simulink library "csu_mhn_miru_hardware_noise_lib"  (R2015b)
settings: Solver=ode45  SolverMode=SingleTasking  StartTime=0.0  StopTime=10.0  RelTol=1e-3
values from neighbouring files (symbols this model uses):
  mhn_accel_range = 3*9.81    (= 29.43)    [csu_mhn_miru_hardware_noise_init.m]
  mhn_accel_SF = 300/1e6    (= 0.0003)    [csu_mhn_miru_hardware_noise_init.m]
  mhn_correlation_time = 100    [csu_mhn_miru_hardware_noise_init.m]
  mhn_dt = sim_time_step_size    [csu_mhn_miru_hardware_noise_init.m]
  mhn_gyro_g_sensitive = 2.471e-08 * [1 1 1]'    [csu_mhn_miru_hardware_noise_init.m]
  mhn_gyro_range = 250*pi/180    (= 4.36332312999)    [csu_mhn_miru_hardware_noise_init.m]
  mhn_gyro_SF = 100/1e6    (= 0.0001)    [csu_mhn_miru_hardware_noise_init.m]
  mhn_gyro_vibe_sensitive = 5.04e-09 * [1 1 1]'    [csu_mhn_miru_hardware_noise_init.m]
libraries: util_common_lib x7, util_info_lib x1
settings Model: Creator=hcannon  LastModifiedBy=Mark Agbayani
settings DataIOCC: SaveFormat=Array  SignalLoggingSaveFormat=ModelDataLogs
settings OptimizationCC: BlockReduction=off  BooleanDataType=off  ExpressionDepthLimit=2147483647
settings DebuggingCC: SaveWithParameterizedLinksMsg=none  UnderspecifiedInitializationDetection=Classic  MergeDetectMultiDrivingBlocksExec=none  SignalResolutionControl=TryResolveAllWithWarning  FcnCallInpInsideContextMsg=EnableAllAsWarning  StateNameClashWarn=warning  StrictBusMsg=Warning
settings HardwareCC: ProdBitPerPointer=32  ProdLargestAtomicFloat=None  ProdIntDivRoundTo=Undefined  ProdEndianess=Unspecified  ProdWordSize=32  ProdHWDeviceType=32-bit Generic  TargetUnknown=on
settings GRTTargetCC: GeneratePreprocessorConditionals=Disable all  CombineOutputUpdateFcns=off  GRTInterface=on
settings ConfigComp: CovModelRefEnable=Off  CovSFcnEnable=off

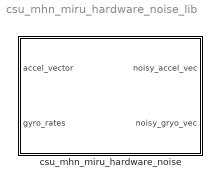
== system csu_mhn_miru_hardware_noise_lib ==
  csu_mhn_miru_hardware_noise : Subsystem

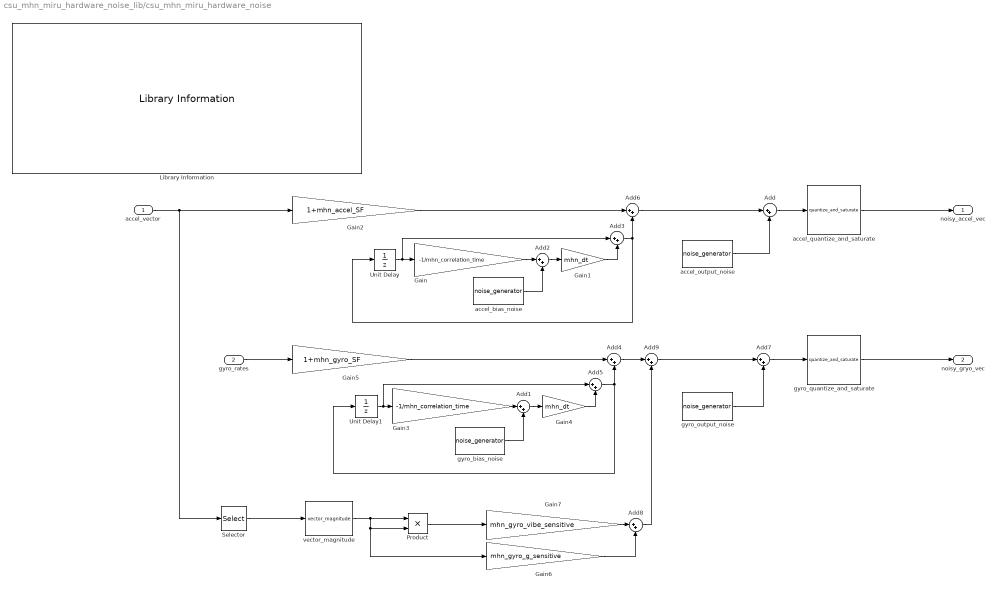
== system csu_mhn_miru_hardware_noise_lib/csu_mhn_miru_hardware_noise ==
  accel_vector : Inport
  gyro_rates : Inport  Port=2
  Add{,1..9} (10 alike) : Sum  Inputs=|++
  Gain : Gain  Gain=-1/mhn_correlation_time
  Gain1 : Gain  Gain=mhn_dt
  Gain2 : Gain  Gain=1+mhn_accel_SF
  Gain3 : Gain  Gain=-1/mhn_correlation_time
  Gain4 : Gain  Gain=mhn_dt
  Gain5 : Gain  Gain=1+mhn_gyro_SF
  Gain6 : Gain  Gain=mhn_gyro_g_sensitive
  Gain7 : Gain  Gain=mhn_gyro_vibe_sensitive
  Library Information : util_info_lib/Library Information  owner='escrane'
  Product : Product  RndMeth=Zero
  Selector : Selector  InputPortWidth=8  IndexOptions=Index vector (dialog)  Indices=mhn_three_axis_index  OutputSizes=1
  Unit Delay : UnitDelay  SampleTime=-1
  Unit Delay1 : UnitDelay  SampleTime=-1
  accel_bias_noise : util_common_lib/noise_generator  std_dev=mhn_accel_bias_noise_v  bias=mhn_accel_bias_bias_v  seed=mhn_accel_bias_seed_v  on=mhn_accel_bias_noise_on  sample_time=sim_time_step_size
  accel_output_noise : util_common_lib/noise_generator  std_dev=mhn_accel_noise_v  bias=mhn_accel_bias_v  seed=mhn_accel_seed_v  on=mhn_accel_noise_on  sample_time=sim_time_step_size
  accel_quantize_and_saturate : util_common_lib/quantize_and_saturate  RES=mhn_accel_sensitivity  OPER=truncate  out_min=-mhn_accel_range  out_max=mhn_accel_range
  gyro_bias_noise : util_common_lib/noise_generator  std_dev=mhn_gyro_bias_noise_v  bias=mhn_gyro_bias_bias_v  seed=mhn_gyro_bias_seed_v  on=mhn_gyro_bias_noise_on  sample_time=sim_time_step_size
  gyro_output_noise : util_common_lib/noise_generator  std_dev=mhn_gyro_noise_v  bias=mhn_gyro_bias_v  seed=mhn_gyro_seed_v  on=mhn_gyro_noise_on  sample_time=sim_time_step_size
  gyro_quantize_and_saturate : util_common_lib/quantize_and_saturate  RES=mhn_gyro_sensitivity  OPER=truncate  out_min=-mhn_gyro_range  out_max=mhn_gyro_range
  vector_magnitude : util_common_lib/vector_magnitude  SystemSampleTime=-1
  noisy_accel_vec : Outport
  noisy_gryo_vec : Outport  Port=2
  wires:
  Add8/1 -> Add9/2
  Add9/1 -> Add7/1
  Add4/1 -> Add9/1
  Gain6/1 -> Add8/2
  Gain7/1 -> Add8/1
  Product/1 -> Gain7/1
  vector_magnitude/1 -> Gain6/1, Product/2, Product/1
  Add6/1 -> Add/1
  Gain2/1 -> Add6/1
  Gain5/1 -> Add4/1
  Add/1 -> accel_quantize_and_saturate/1
  accel_quantize_and_saturate/1 -> noisy_accel_vec/1
  gyro_quantize_and_saturate/1 -> noisy_gryo_vec/1
  accel_output_noise/1 -> Add/2
  Add2/1 -> Gain1/1
  Gain1/1 -> Add3/2
  Unit Delay/1 -> Gain/1, Add3/1
  Add3/1 -> Add6/2, Unit Delay/1
  accel_vector/1 -> Selector/1, Gain2/1
  Gain/1 -> Add2/1
  accel_bias_noise/1 -> Add2/2
  Add1/1 -> Gain4/1
  Gain4/1 -> Add5/2
  Unit Delay1/1 -> Gain3/1, Add5/1
  Add5/1 -> Unit Delay1/1, Add4/2
  gyro_rates/1 -> Gain5/1
  Gain3/1 -> Add1/1
  gyro_bias_noise/1 -> Add1/2
  Add7/1 -> gyro_quantize_and_saturate/1
  gyro_output_noise/1 -> Add7/2
  Selector/1 -> vector_magnitude/1
